simulink model "rRegenPaddle"  (R2024b)
settings: configuration reference "STM32H7_Config" (kept outside this file)
undefined symbols (not defined in the file): rRegenPaddleCalHigh, rRegenPaddleCalLow, VRegenPaddle1HighSample, VRegenPaddle1LowSample, VRegenPaddle2HighSample, VRegenPaddle2LowSample
libraries: simulink x1
settings Model: DataDictionary=Master_Dictionary.sldd  EnableAccessToBaseWorkspace=off  Creator=torni  LastModifiedBy=William
settings ConfigSetRef: SourceName=STM32H7_Config

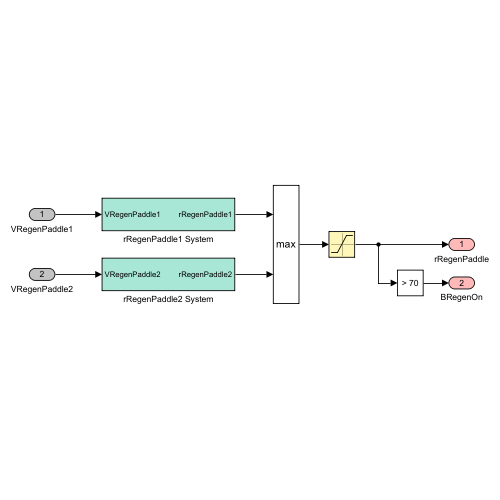
[thumbnail: Simulink's stored preview of the top-level diagram]
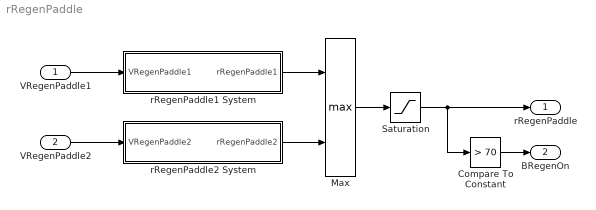
== system rRegenPaddle ==
  VRegenPaddle1 : Inport  OutDataTypeStr=double
  VRegenPaddle2 : Inport  Port=2  OutDataTypeStr=double
  Compare To Constant : simulink/Logic and Bit Operations/Compare To Constant  relop=>  const=70  OutDataTypeStr=boolean
  Max : MinMax  Function=max  Inputs=2
  Saturation : Saturate  UpperLimit=100  LowerLimit=0
  rRegenPaddle1 System : Subsystem
  rRegenPaddle2 System : Subsystem
  rRegenPaddle : Outport  OutDataTypeStr=double  VectorParamsAs1DForOutWhenUnconnected=off
  "BRegenOn " : Outport  Port=2  OutDataTypeStr=boolean  VectorParamsAs1DForOutWhenUnconnected=off
  wires:
  Saturation/1 -> Compare To Constant/1, rRegenPaddle/1
  Compare To Constant/1 -> "BRegenOn "/1
  Max/1 -> Saturation/1
  VRegenPaddle2/1 -> rRegenPaddle2 System/1(VRegenPaddle2)
  VRegenPaddle1/1 -> rRegenPaddle1 System/1(VRegenPaddle1)
  rRegenPaddle2 System/1(rRegenPaddle2) -> Max/2
  rRegenPaddle1 System/1(rRegenPaddle1) -> Max/1

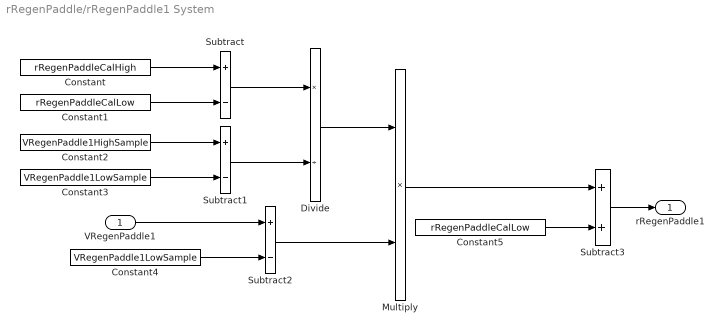
== system rRegenPaddle/rRegenPaddle1 System ==
  VRegenPaddle1 : Inport  OutDataTypeStr=double
  Constant : Constant  Value=rRegenPaddleCalHigh
  Constant1 : Constant  Value=rRegenPaddleCalLow
  Constant2 : Constant  Value=VRegenPaddle1HighSample
  Constant3 : Constant  Value=VRegenPaddle1LowSample
  Constant4 : Constant  Value=VRegenPaddle1LowSample
  Constant5 : Constant  Value=rRegenPaddleCalLow
  Divide : Product  Inputs=*/
  Multiply : Product
  Subtract : Sum  Inputs=+-
  Subtract1 : Sum  Inputs=+-
  Subtract2 : Sum  Inputs=+-
  Subtract3 : Sum
  rRegenPaddle1 : Outport  OutDataTypeStr=double  VectorParamsAs1DForOutWhenUnconnected=off
  wires:
  VRegenPaddle1/1 -> Subtract2/1
  Subtract1/1 -> Divide/2
  Constant4/1 -> Subtract2/2
  Constant5/1 -> Subtract3/2
  Divide/1 -> Multiply/1
  Subtract3/1 -> rRegenPaddle1/1
  Constant3/1 -> Subtract1/2
  Multiply/1 -> Subtract3/1
  Constant/1 -> Subtract/1
  Constant2/1 -> Subtract1/1
  Subtract2/1 -> Multiply/2
  Subtract/1 -> Divide/1
  Constant1/1 -> Subtract/2

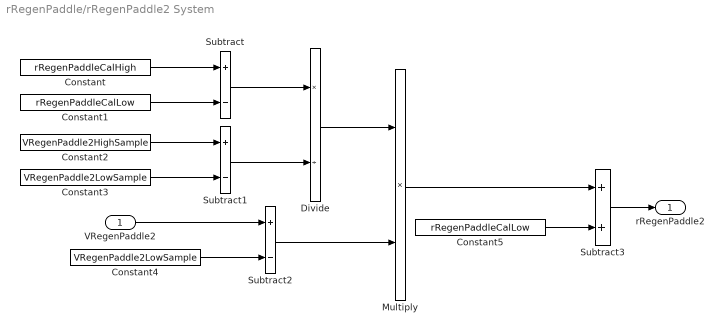
== system rRegenPaddle/rRegenPaddle2 System ==
  VRegenPaddle2 : Inport  OutDataTypeStr=double
  Constant : Constant  Value=rRegenPaddleCalHigh
  Constant1 : Constant  Value=rRegenPaddleCalLow
  Constant2 : Constant  Value=VRegenPaddle2HighSample
  Constant3 : Constant  Value=VRegenPaddle2LowSample
  Constant4 : Constant  Value=VRegenPaddle2LowSample
  Constant5 : Constant  Value=rRegenPaddleCalLow
  Divide : Product  Inputs=*/
  Multiply : Product
  Subtract : Sum  Inputs=+-
  Subtract1 : Sum  Inputs=+-
  Subtract2 : Sum  Inputs=+-
  Subtract3 : Sum
  rRegenPaddle2 : Outport  OutDataTypeStr=double  VectorParamsAs1DForOutWhenUnconnected=off
  wires:
  Constant1/1 -> Subtract/2
  Subtract/1 -> Divide/1
  Subtract2/1 -> Multiply/2
  Constant2/1 -> Subtract1/1
  Constant/1 -> Subtract/1
  Multiply/1 -> Subtract3/1
  Constant3/1 -> Subtract1/2
  Subtract3/1 -> rRegenPaddle2/1
  Divide/1 -> Multiply/1
  Constant5/1 -> Subtract3/2
  Constant4/1 -> Subtract2/2
  Subtract1/1 -> Divide/2
  VRegenPaddle2/1 -> Subtract2/1
